simulink model "Sim_Multi"  (R2023a)
settings: Solver=FixedStepAuto  StartTime=0.0  StopTime=20  FixedStep=t_sim  MaxStep=t_control  RelTol=1e-5  EnableMultiTasking=on
InitFcn:
  | %--------------------------------------------------------------------------
  | %% Multirotor Dynamic Simulation Environment for the Testing of GNC Algorithms
  | % This simulation is part of the Master's thesis titled
  | % "A Modular Simulation Environment for the Improved Dynamic Simulation of
  | % Multirotor Unmanned Aerial Vehicles",
  | % submitted to the University of Illinois at Urbana-Champaign in May 2016.
  | % The thesis itself can be found here: http://hdl.handle.net/2142/90660
  | % Jan Vervoorst, vervoors@illinois.edu
  | % University of Illinois 2015/16
  | %--------------------------------------------------------------------------
  | %% Initialization routine for the Simulink simulation file Sim_Multi.slx
  | %--------------------------------------------------------------------------
  | clear all;close all;clc
  | %--------------------------------------------------------------------------
  | t_control = 1/500;          % Controller/state estimation frequency 500Hz [s]
  | t_sim = t_control/2;        % Simulation frequency 1000Hz [s]
  | sim_time = 10.0;            % Duration of simulation [sec]
  | r2d = 180/pi;               % Conversion factor radians to degrees [deg/rad]
  | d2r = pi/180;               % Conversion factor degrees to radians [rad/deg]
  | g = 9.80665;                % Acceleration of gravity [m/s^2]
  | rpm2radpersec = 2*pi/60;    % Conversion factor RPM to rad/sec [rad/(s*rpm)]
  | rho = 1.225;                % Density of air [kg/m^3]
  | %--------------------------------------------------------------------------
  | %%%%%%%%%%%%%%%%%%%%%%%%%%%%%%%%%%%%%%%%%%%%%%%%%%%%%%%%%%%%%%%%%%%%%%%%%%%
  | %               Quad specific configuration parameters                    %
  | %%%%%%%%%%%%%%%%%%%%%%%%%%%%%%%%%%%%%%%%%%%%%%%%%%%%%%%%%%%%%%%%%%%%%%%%%%%
  | % The coordinate system used in this model is defined as follows:
  | % X: pointing forward, Roll axis
  | % Y: pointing to the right, Pitch axis
  | % Z: pointing down, Yaw axis
  | % To define the geometry of the airframe, the following convention is used:
  | % - the base airframe is assumed to be somewhat symmetric
  | % - the CoG for the base airframe coincides with the geometric center in X/Y plane (but is shifted along Z axis)
  | % - the motor arm length in X/Y plane is defined as the distance to the geometric center of the base airframe
  | % - motor thrust is generated at the prop, which is offset a distance (along Z) from the geometric center
  | % - motor thrust vector may be misaligned from purely Z direction, so a set of rotation angles is given for each motor
  | % - real position of CoG is given as a position vector from geometric center
  | % - everything is expressed in body coordinate system described above
  | %%%%%%%%%%%%%%%%%%%%%%%%%%%%%%%%%%%%%%%%%%%%%%%%%%%%%%%%%%%%%%%%%%%%%%%%%%%
  | Noise_flag = 0;                 % Set to 1 for sensor/estimation noise, to 0 for no noise
  | Coriolis_correction = 1;        % Set to 1 to cancel omega x (J*omega) term in control law, 0 if not
  | Dyn_thrust = 1;                 % Set to 1 to engage dynamic thrust effects, to 0 to disengage
  | Blade_flapping = 1;             % Set to 1 to engage blade flapping effects, to 0 to disengage
  | %%%%%%%%%%%%%%%%%%%%%%%%%%%%%%%%
  | % Initial conditions
  | Att_init = [0;0;0] * d2r;       % Initial airframe attitude in Euler angles Roll/Pitch/Yaw for 6DOF block [deg]
  | omega_init = [0;0;0];           % Initial angular rates in Body frame for 6DOF block [rad/s]
  | Vb_init = [0;0;0];              % Initial velocity in Body frame for 6DOF block [m/s]
  | Xi_init = [0;0;0];              % Initial position in Inertial frame for 6DOF block [m]
  | rpm_init = 3104.5025852;        % Initial motor speed [rpm]
  | q_init = rpy2quat(Att_init);    % Compute the initial attitude quaternion
  | R_IB_init = rpy2rot(Att_init);  % Compute the initial rotation matrix R_IB
  | Vi_init = R_IB_init' * Vb_init; % Compute the initial velocity in Inertial axes
  | %%%%%%%%%%%%%%%%%%%%%%%%%%%%%%%%
  | % Parameters for aerodynamic drag computation
  | a = 0.060;                      % Surface area of airframe visible along the Body x axis [m^2]
  | b = 0.060;                      % Surface area of airframe visible along the Body y axis [m^2]
  | c = 0.060;                      % Surface area of airframe visible along the Body z axis [m^2]
  | C_D = 0.40;                     % Drag coefficient [dimensionless]
  | Surface_params = [a;b;c];       % Combine the surface area parameters
  | ... (+145 lines)
undefined symbols (not defined in the file or in its folder): DiscIntNeverNeededParam, rpy2quat, thrust2rpm
libraries: simulink x20
(part 2 of 4)

== system Sim_Multi/State Estimation, Sensors, Noise/State estimation/Normalize ==
  Input : Inport
  Divide : Product  Inputs=*/
  norm : Subsystem
  Output : Outport
  wires:
  Input/1 -> Divide/1, norm/1(u)
  norm/1(||u||) -> Divide/2
  Divide/1 -> Output/1

== system Sim_Multi/State Estimation, Sensors, Noise/State estimation/Quat noise ==
  Band-Limited White Noise : simulink/Sources/Band-Limited White Noise  Cov=t_sim*57.3*57.3/10000  Ts=t_sim*30  seed=[23099]
  Constant : Constant  Value=Noise_flag
  Constant1 : Constant  Value=0
  Gain2 : Gain  Gain=0.1
  Rate Transition1 : RateTransition  OutPortSampleTime=t_sim
  Switch : Switch  Criteria=u2 > Threshold  SaturateOnIntegerOverflow=off  InputSameDT=off
  Noise : Outport
  wires:
  Band-Limited White Noise/1 -> Gain2/1
  Switch/1 -> Noise/1
  Constant/1 -> Switch/2
  Constant1/1 -> Switch/3
  Gain2/1 -> Rate Transition1/1
  Rate Transition1/1 -> Switch/1

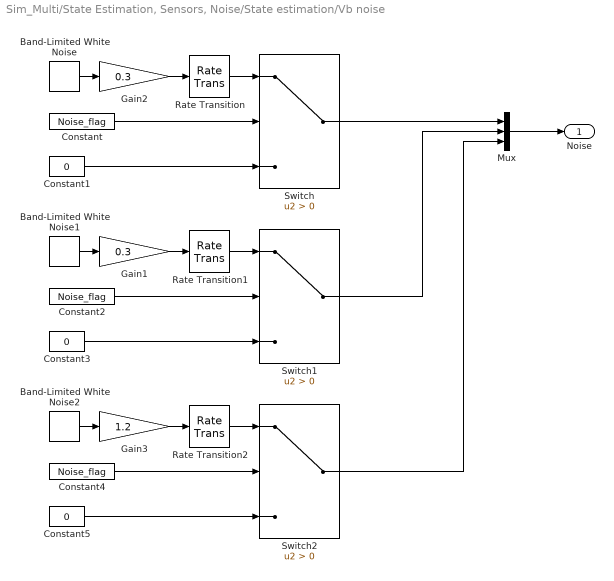
== system Sim_Multi/State Estimation, Sensors, Noise/State estimation/Vb noise ==
  Band-Limited White Noise : simulink/Sources/Band-Limited White Noise  Cov=t_sim*57.3*57.3/10000  Ts=t_sim*10  seed=[21234]
  Band-Limited White Noise1 : simulink/Sources/Band-Limited White Noise  Cov=t_sim*57.3*57.3/10000  Ts=t_sim*10  seed=[21234]
  Band-Limited White Noise2 : simulink/Sources/Band-Limited White Noise  Cov=t_sim*57.3*57.3/10000  Ts=t_sim*10  seed=[21234]
  Constant : Constant  Value=Noise_flag
  Constant1 : Constant  Value=0
  Constant2 : Constant  Value=Noise_flag
  Constant3 : Constant  Value=0
  Constant4 : Constant  Value=Noise_flag
  Constant5 : Constant  Value=0
  Gain1 : Gain  Gain=0.3
  Gain2 : Gain  Gain=0.3
  Gain3 : Gain  Gain=1.2
  Mux : Mux  Inputs=3
  Rate Transition : RateTransition  OutPortSampleTime=t_sim
  Rate Transition1 : RateTransition  OutPortSampleTime=t_sim
  Rate Transition2 : RateTransition  OutPortSampleTime=t_sim
  Switch : Switch  Criteria=u2 > Threshold  SaturateOnIntegerOverflow=off  InputSameDT=off
  Switch1 : Switch  Criteria=u2 > Threshold  SaturateOnIntegerOverflow=off  InputSameDT=off
  Switch2 : Switch  Criteria=u2 > Threshold  SaturateOnIntegerOverflow=off  InputSameDT=off
  Noise : Outport
  wires:
  Band-Limited White Noise/1 -> Gain2/1
  Constant/1 -> Switch/2
  Constant1/1 -> Switch/3
  Gain2/1 -> Rate Transition/1
  Rate Transition/1 -> Switch/1
  Switch/1 -> Mux/1
  Mux/1 -> Noise/1
  Band-Limited White Noise1/1 -> Gain1/1
  Constant2/1 -> Switch1/2
  Constant3/1 -> Switch1/3
  Gain1/1 -> Rate Transition1/1
  Rate Transition1/1 -> Switch1/1
  Band-Limited White Noise2/1 -> Gain3/1
  Constant4/1 -> Switch2/2
  Constant5/1 -> Switch2/3
  Gain3/1 -> Rate Transition2/1
  Rate Transition2/1 -> Switch2/1
  Switch1/1 -> Mux/2
  Switch2/1 -> Mux/3

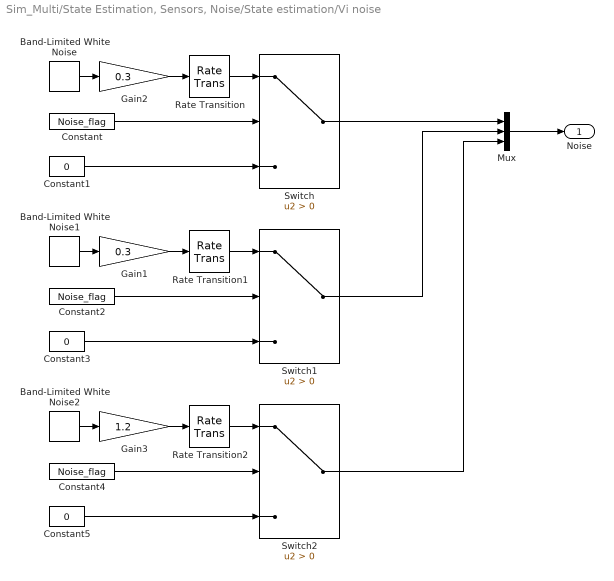
== system Sim_Multi/State Estimation, Sensors, Noise/State estimation/Vi noise ==
  Band-Limited White Noise : simulink/Sources/Band-Limited White Noise  Cov=t_sim*57.3*57.3/10000  Ts=t_sim*10  seed=[23888]
  Band-Limited White Noise1 : simulink/Sources/Band-Limited White Noise  Cov=t_sim*57.3*57.3/10000  Ts=t_sim*10  seed=[23888]
  Band-Limited White Noise2 : simulink/Sources/Band-Limited White Noise  Cov=t_sim*57.3*57.3/10000  Ts=t_sim*10  seed=[23888]
  Constant : Constant  Value=Noise_flag
  Constant1 : Constant  Value=0
  Constant2 : Constant  Value=Noise_flag
  Constant3 : Constant  Value=0
  Constant4 : Constant  Value=Noise_flag
  Constant5 : Constant  Value=0
  Gain1 : Gain  Gain=0.3
  Gain2 : Gain  Gain=0.3
  Gain3 : Gain  Gain=1.2
  Mux : Mux  Inputs=3
  Rate Transition : RateTransition  OutPortSampleTime=t_sim
  Rate Transition1 : RateTransition  OutPortSampleTime=t_sim
  Rate Transition2 : RateTransition  OutPortSampleTime=t_sim
  Switch : Switch  Criteria=u2 > Threshold  SaturateOnIntegerOverflow=off  InputSameDT=off
  Switch1 : Switch  Criteria=u2 > Threshold  SaturateOnIntegerOverflow=off  InputSameDT=off
  Switch2 : Switch  Criteria=u2 > Threshold  SaturateOnIntegerOverflow=off  InputSameDT=off
  Noise : Outport
  wires:
  Band-Limited White Noise/1 -> Gain2/1
  Constant/1 -> Switch/2
  Constant1/1 -> Switch/3
  Gain2/1 -> Rate Transition/1
  Rate Transition/1 -> Switch/1
  Switch/1 -> Mux/1
  Mux/1 -> Noise/1
  Band-Limited White Noise1/1 -> Gain1/1
  Constant2/1 -> Switch1/2
  Constant3/1 -> Switch1/3
  Gain1/1 -> Rate Transition1/1
  Rate Transition1/1 -> Switch1/1
  Band-Limited White Noise2/1 -> Gain3/1
  Constant4/1 -> Switch2/2
  Constant5/1 -> Switch2/3
  Gain3/1 -> Rate Transition2/1
  Rate Transition2/1 -> Switch2/1
  Switch1/1 -> Mux/2
  Switch2/1 -> Mux/3

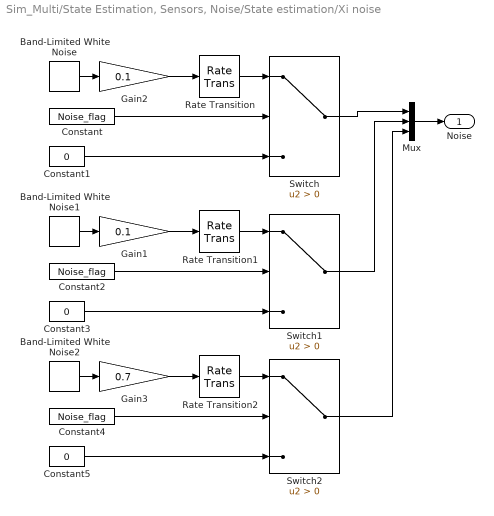
== system Sim_Multi/State Estimation, Sensors, Noise/State estimation/Xi noise ==
  Band-Limited White Noise : simulink/Sources/Band-Limited White Noise  Cov=t_sim*57.3*57.3/10000  Ts=t_sim*20  seed=[23559]
  Band-Limited White Noise1 : simulink/Sources/Band-Limited White Noise  Cov=t_sim*57.3*57.3/10000  Ts=t_sim*20  seed=[23559]
  Band-Limited White Noise2 : simulink/Sources/Band-Limited White Noise  Cov=t_sim*57.3*57.3/10000  Ts=t_sim*20  seed=[23559]
  Constant : Constant  Value=Noise_flag
  Constant1 : Constant  Value=0
  Constant2 : Constant  Value=Noise_flag
  Constant3 : Constant  Value=0
  Constant4 : Constant  Value=Noise_flag
  Constant5 : Constant  Value=0
  Gain1 : Gain  Gain=0.1
  Gain2 : Gain  Gain=0.1
  Gain3 : Gain  Gain=0.7
  Mux : Mux  Inputs=3
  Rate Transition : RateTransition  OutPortSampleTime=t_sim
  Rate Transition1 : RateTransition  OutPortSampleTime=t_sim
  Rate Transition2 : RateTransition  OutPortSampleTime=t_sim
  Switch : Switch  Criteria=u2 > Threshold  SaturateOnIntegerOverflow=off  InputSameDT=off
  Switch1 : Switch  Criteria=u2 > Threshold  SaturateOnIntegerOverflow=off  InputSameDT=off
  Switch2 : Switch  Criteria=u2 > Threshold  SaturateOnIntegerOverflow=off  InputSameDT=off
  Noise : Outport
  wires:
  Band-Limited White Noise/1 -> Gain2/1
  Constant/1 -> Switch/2
  Constant1/1 -> Switch/3
  Gain2/1 -> Rate Transition/1
  Mux/1 -> Noise/1
  Switch/1 -> Mux/1
  Band-Limited White Noise1/1 -> Gain1/1
  Constant2/1 -> Switch1/2
  Constant3/1 -> Switch1/3
  Gain1/1 -> Rate Transition1/1
  Band-Limited White Noise2/1 -> Gain3/1
  Constant4/1 -> Switch2/2
  Constant5/1 -> Switch2/3
  Gain3/1 -> Rate Transition2/1
  Switch1/1 -> Mux/2
  Switch2/1 -> Mux/3
  Rate Transition/1 -> Switch/1
  Rate Transition1/1 -> Switch1/1
  Rate Transition2/1 -> Switch2/1

== system Sim_Multi/multirotor/6DOF model/Body to Inertial ==
  V_b : Inport
  DCM_ib : Inport  Port=2
  Math Function2 : Math  Operator=transpose  SignedPower=on
  Product : Product  Multiplication=Matrix(*)
  Reshape : Reshape  OutputDimensionality=Column vector (2-D)
  Reshape1 : Reshape  OutputDimensionality=Column vector (2-D)
  V_i : Outport
  wires:
  Reshape/1 -> Product/2
  Product/1 -> Reshape1/1
  DCM_ib/1 -> Math Function2/1
  Reshape1/1 -> V_i/1
  V_b/1 -> Reshape/1
  Math Function2/1 -> Product/1  "DCM_bi"

== system Sim_Multi/multirotor/6DOF model/Body to Inertial1 ==
  a_b : Inport
  DCM_ib : Inport  Port=2
  Math Function2 : Math  Operator=transpose  SignedPower=on
  Product : Product  Multiplication=Matrix(*)
  Reshape : Reshape  OutputDimensionality=Column vector (2-D)
  Reshape1 : Reshape  OutputDimensionality=Column vector (2-D)
  a_i : Outport
  wires:
  Reshape/1 -> Product/2
  Product/1 -> Reshape1/1
  DCM_ib/1 -> Math Function2/1
  Reshape1/1 -> a_i/1
  a_b/1 -> Reshape/1
  Math Function2/1 -> Product/1  "DCM_bi"

== system Sim_Multi/multirotor/6DOF model/Calculate omega_dot ==
  omega [rad/s] : Inport
  Inertia [kgm^2] : Inport  Port=2
  Moments [Nm] : Inport  Port=3
  Cross Product omega x (J * omega) : Subsystem
  Product : Product  Inputs=/*  Multiplication=Matrix(*)
  Reshape : Reshape  OutputDimensionality=Column vector (2-D)
  "Reshape " : Reshape  OutputDimensionality=Column vector (2-D)
  Subsystem : Subsystem
  Sum1 : Sum  Inputs=-+|
  omega_dot [rad/s^2] : Outport
  wires:
  Inertia [kgm^2]/1 -> Product/1, Subsystem/2(J)
  omega [rad/s]/1 -> Cross Product omega x (J * omega)/1(omega), Subsystem/1(omega)
  Subsystem/1(J * omega) -> Cross Product omega x (J * omega)/2(J * omega)
  Cross Product omega x (J * omega)/1(omega x (J * omega)) -> Reshape/1
  Product/1 -> "Reshape "/1
  "Reshape "/1 -> omega_dot [rad/s^2]/1
  Moments [Nm]/1 -> Sum1/2
  Reshape/1 -> Sum1/1
  Sum1/1 -> Product/2

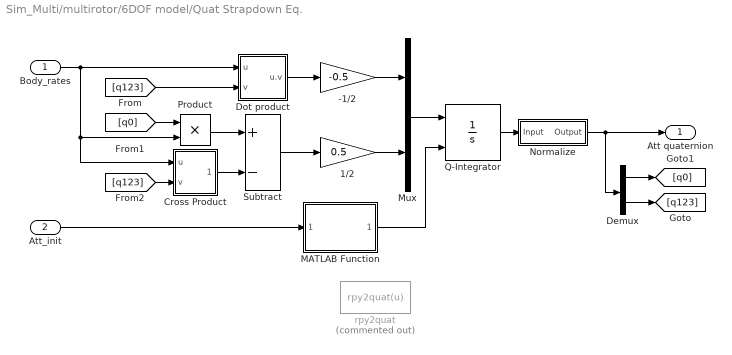
== system Sim_Multi/multirotor/6DOF model/Quat Strapdown Eq. ==
  Body_rates : Inport
  Att_init : Inport  Port=2
  -1/2 : Gain  Gain=-0.5
  1/2 : Gain  Gain=0.5
  Cross Product : Subsystem
  Demux : Demux  Outputs=[1 3]
  Dot product : Subsystem
  MATLAB Function : MATLAB Function  TreatAsAtomicUnit=on
  Mux : Mux  Inputs=[1 3]
  Normalize : Subsystem
  Product : Product  RndMeth=Zero
  Q-Integrator : Integrator  InitialConditionSource=external  InitialCondition=[1 0 0 0]
  Subtract : Sum  Inputs=+-
  rpy2quat : MATLABFcn  Commented=on  MATLABFcn=rpy2quat(u)  OutputDimensions=4
  Att quaternion : Outport
  wires:
  Dot product/1(u.v) -> -1/2/1
  -1/2/1 -> Mux/1
  Body_rates/1 -> Dot product/1(u), Cross Product/1(u), Product/2
  Q-Integrator/1 -> Normalize/1(Input)
  [q123] -> Dot product/2(v)
  Product/1 -> Subtract/1
  Cross Product/1(u x v) -> Subtract/2
  [q0] -> Product/1
  [q123] -> Cross Product/2(v)
  Subtract/1 -> 1/2/1
  1/2/1 -> Mux/2
  Demux/1 -> [q0]
  Demux/2 -> [q123]
  Normalize/1(Output) -> Demux/1, Att quaternion/1
  Mux/1 -> Q-Integrator/1
  MATLAB Function/1(quat_output) -> Q-Integrator/2
  Att_init/1 -> MATLAB Function/1(quat_input)

== system Sim_Multi/multirotor/6DOF model/Quat to Euler ==
  Quaternion q : Inport
  Fcn : Fcn  Expr=2*(u(3)*u(4)+u(1)*u(2))
  Fcn1 : Fcn  Expr=2*(u(2)*u(4)-u(1)*u(3))
  Fcn2 : Fcn  Expr=2*(u(2)*u(3)+u(1)*u(4))
  Fcn3 : Fcn  Expr=u(1)*u(1)-u(2)*u(2)-u(3)*u(3)+u(4)*u(4)
  Fcn4 : Fcn  Expr=u(1)*u(1)+u(2)*u(2)-u(3)*u(3)-u(4)*u(4)
  Gain : Gain  Gain=-1
  Reshape : Reshape  OutputDimensionality=Column vector (2-D)
  Trigonometric Function : Trigonometry  Operator=asin
  Trigonometric Function1 : Trigonometry  Operator=atan2
  Trigonometric Function2 : Trigonometry  Operator=atan2
  Vector Concatenate : Concatenate  NumInputs=3
  Euler [rad] : Outport
  wires:
  Fcn1/1 -> Trigonometric Function/1
  Trigonometric Function/1 -> Gain/1
  Fcn/1 -> Trigonometric Function1/1
  Fcn3/1 -> Trigonometric Function1/2
  Fcn2/1 -> Trigonometric Function2/1
  Fcn4/1 -> Trigonometric Function2/2
  Trigonometric Function1/1 -> Vector Concatenate/1
  Gain/1 -> Vector Concatenate/2
  Trigonometric Function2/1 -> Vector Concatenate/3
  Quaternion q/1 -> Fcn4/1, Fcn2/1, Fcn/1, Fcn3/1, Fcn1/1
  Vector Concatenate/1 -> Reshape/1
  Reshape/1 -> Euler [rad]/1

== system Sim_Multi/multirotor/6DOF model/Quat to Rotation Matrix ==
  Quaternion q : Inport
  Subsystem : Subsystem
  Subsystem1 : Subsystem
  Subsystem2 : Subsystem
  Subsystem3 : Subsystem
  Subsystem4 : Subsystem
  Subsystem5 : Subsystem
  Subsystem6 : Subsystem
  Subsystem7 : Subsystem
  Subsystem8 : Subsystem
  Subsystem9 : Subsystem
  DCM_ib : Outport
  wires:
  Quaternion q/1 -> Subsystem2/1(q), Subsystem8/1(q), Subsystem7/1(q), Subsystem6/1(q), Subsystem1/1(q), Subsystem5/1(q), Subsystem4/1(q), Subsystem3/1(q), Subsystem/1(q)
  Subsystem/1(C_11) -> Subsystem9/1(C_11)
  Subsystem3/1(C_12) -> Subsystem9/2(C_12)
  Subsystem4/1(C_13) -> Subsystem9/3(C_13)
  Subsystem5/1(C_21) -> Subsystem9/4(C_21)
  Subsystem1/1(C_22) -> Subsystem9/5(C_22)
  Subsystem2/1(C_33) -> Subsystem9/9(C_33)
  Subsystem8/1(C_32) -> Subsystem9/8(C_32)
  Subsystem7/1(C_31) -> Subsystem9/7(C_31)
  Subsystem6/1(C_23) -> Subsystem9/6(C_23)
  Subsystem9/1(DCM_ib) -> DCM_ib/1

== system Sim_Multi/multirotor/6DOF model/omega x V_b ==
  V_b : Inport
  omega : Inport  Port=2
  Subsystem : Subsystem
  Subsystem1 : Subsystem
  Sum : Sum  Inputs=+|-
  omega x V_b : Outport
  wires:
  Sum/1 -> omega x V_b/1
  omega/1 -> Subsystem1/1(u), Subsystem/1(u)
  V_b/1 -> Subsystem/2(v), Subsystem1/2(v)
  Subsystem/1(Positive elements) -> Sum/1
  Subsystem1/1(Negative elements) -> Sum/2

== system Sim_Multi/multirotor/Force//Moment computation/Compute aerodynamic drag of the airframe in Body axes ==
  note: Aerodynamic drag force acting on the airframe
      | The assumption is that the surface area of the airframe from different directions
      | can be described by an ellipsoid. Then the 'acting 'surface area is in the direction
      | of the airspeed vector and can be computed by scaling the airspeed vector so that
      | it points onto the surface of the ellipsoid.
  6DOF dynamics : Inport
  Dynamic parameters : Inport  Port=2
  Aerodynamic drag force : Subsystem
  Bus Selector2 : BusSelector  OutputSignals=V_b,DCM_ib
  Bus Selector3 : BusSelector  OutputSignals=Wind_i,Surface_params
  Total airspeed (Body axes) : Subsystem
  Drag force : Outport
  wires:
  Aerodynamic drag force/1(Drag force (Body axes)) -> Drag force/1
  6DOF dynamics/1 -> Bus Selector2/1
  Dynamic parameters/1 -> Bus Selector3/1
  Bus Selector3/2 -> Aerodynamic drag force/2(Surface_params)  "<Surface_params>"
  Bus Selector2/1 -> Total airspeed (Body axes)/1(V_b)  "<V_b>"
  Bus Selector2/2 -> Total airspeed (Body axes)/2(DCM_ib)  "<DCM_ib>"
  Bus Selector3/1 -> Total airspeed (Body axes)/3(Wind_i)  "<Wind_i>"
  Total airspeed (Body axes)/1(Airspeed (Body)) -> Aerodynamic drag force/1(Airspeed (Body axes))

== system Sim_Multi/multirotor/Force//Moment computation/Compute force of gravity in Body axes ==
  note: Force of gravity acting on the airframe
  6DOF dynamics : Inport
  Dynamic parameters : Inport  Port=2
  Bus Selector : BusSelector  OutputSignals=DCM_ib
  Bus Selector1 : BusSelector  OutputSignals=mass_real
  Gravity (Inertial axes) : Constant  Value=[0;0;g]
  Product : Product  Multiplication=Matrix(*)  InputSameDT=on  SaturateOnIntegerOverflow=on  OutDataTypeStr=Inherit: Same as first input
  Product1 : Product
  Reshape : Reshape  OutputDimensionality=Column vector (2-D)
  Gravity force : Outport
  wires:
  Gravity (Inertial axes)/1 -> Product1/1
  Product1/1 -> Product/2  "Force of gravity (Inertial axes)"
  Product/1 -> Reshape/1  "Force of gravity (Body axes)"
  Reshape/1 -> Gravity force/1
  6DOF dynamics/1 -> Bus Selector/1
  Dynamic parameters/1 -> Bus Selector1/1
  Bus Selector1/1 -> Product1/2  "<mass_real>"
  Bus Selector/1 -> Product/1  "<DCM_ib>"

== system Sim_Multi/multirotor/Force//Moment computation/Forces and moments generated by spinning propellers ==
  note: Computation of forces and moments for each actuator specified in the initialization routine
  RPM_commands : Inport
  Dynamic parameters : Inport  Port=2
  6DOF dynamics : Inport  Port=3
  Bus Selector : BusSelector  OutputSignals=omega,V_b,DCM_ib
  Bus Selector1 : BusSelector  OutputSignals=Wind_i,MotorMatrix_real,CoG_real
  For Each Subsystem : Subsystem  TreatAsAtomicUnit=on
  Reshape : Reshape  OutputDimensionality=Column vector (2-D)
  Sum of Elements : Sum  Inputs=+  CollapseMode=Specified dimension  CollapseDim=2
  Sum of Elements1 : Sum  Inputs=+  CollapseMode=Specified dimension  CollapseDim=2
  To Workspace : ToWorkspace  VariableName=rpm_motor  SaveFormat=Structure With Time  SampleTime=-1
      settings: Save2DSignal=2-D array (concatenate along first dimension)
  Total airspeed (Body axes) : Subsystem
  Motor moments : Outport
  Motor forces : Outport  Port=2
  motor_RPM : Outport  Port=3
  tag scope: RPM_motor=global
  wires:
  For Each Subsystem/1(Motor_force) -> Sum of Elements/1
  For Each Subsystem/2(Motor_moment) -> Sum of Elements1/1
  Sum of Elements/1 -> Motor forces/1
  Sum of Elements1/1 -> Motor moments/1
  RPM_commands/1 -> For Each Subsystem/1(RPM_commands)
  6DOF dynamics/1 -> Bus Selector/1
  Bus Selector/1 -> For Each Subsystem/2(Body_rates)  "<omega>"
  Dynamic parameters/1 -> Bus Selector1/1
  Bus Selector1/2 -> For Each Subsystem/4(MotorMatrix_real)  "<MotorMatrix_real>"
  Bus Selector1/3 -> For Each Subsystem/5(CoG_real)  "<CoG_real>"
  Bus Selector/2 -> Total airspeed (Body axes)/1(V_b)  "<V_b>"
  Bus Selector/3 -> Total airspeed (Body axes)/2(DCM_ib)  "<DCM_ib>"
  Bus Selector1/1 -> Total airspeed (Body axes)/3(Wind_i)  "<Wind_i>"
  Total airspeed (Body axes)/1(Airspeed (Body)) -> For Each Subsystem/3(Airspeed (Body))
  For Each Subsystem/3(RPM_motor) -> Reshape/1
  Reshape/1 -> To Workspace/1, motor_RPM/1, [RPM_motor]

== system Sim_Multi/Controller/Controller Structure/Inner-loop control only/Conversion stick values to rate commands ==
  Sticks/Throttle cmd : Inport
  Constant : Constant  Value=thrust_offset
  Demux8 : Demux  Outputs=[3 1]
  Mux3 : Mux  Inputs=2
  Sum4 : Sum  Inputs=|++
  Unit conversion [stick value] to [N] : Gain  Gain=thrust_gain
  Unit conversion [stick value] to [rad/s] : Gain  Gain=MaxRate_cmd/500
  Rates/Throttle cmd : Outport
  wires:
  Sticks/Throttle cmd/1 -> Demux8/1
  Demux8/1 -> Unit conversion [stick value] to [rad/s]/1
  Unit conversion [stick value] to [N]/1 -> Sum4/1
  Constant/1 -> Sum4/2
  Demux8/2 -> Unit conversion [stick value] to [N]/1  "Throttle cmd"
  Sum4/1 -> Mux3/2  "Throttle command (thrust value)"
  Mux3/1 -> Rates/Throttle cmd/1
  Unit conversion [stick value] to [rad/s]/1 -> Mux3/1

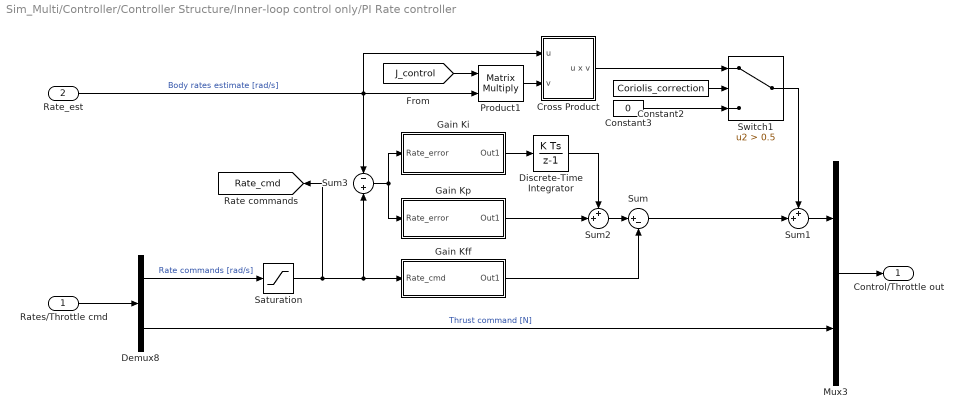
== system Sim_Multi/Controller/Controller Structure/Inner-loop control only/PI Rate controller ==
  Rates/Throttle cmd : Inport
  Rate_est : Inport  Port=2
  Constant2 : Constant  Value=Coriolis_correction
  Constant3 : Constant  Value=0
  Cross Product : Subsystem
  Demux8 : Demux  Outputs=[3 1]
  Discrete-Time Integrator : DiscreteIntegrator  SampleTime=t_control  ICPrevOutput=DiscIntNeverNeededParam  ICPrevScaledInput=DiscIntNeverNeededParam
  Gain Kff : Subsystem
  Gain Ki : Subsystem
  Gain Kp : Subsystem
  Mux3 : Mux  Inputs=2
  Product1 : Product  Multiplication=Matrix(*)  RndMeth=Zero  SampleTime=t_control
  Saturation : Saturate  UpperLimit=MaxRate_cmd  LowerLimit=-MaxRate_cmd
  Sum : Sum  Inputs=|+-
  Sum1 : Sum  Inputs=++|
  Sum2 : Sum  Inputs=++|
  Sum3 : Sum  Inputs=-|+
  Switch1 : Switch  Criteria=u2 > Threshold  Threshold=0.5  SampleTime=t_control  SaturateOnIntegerOverflow=off  InputSameDT=off
  Control/Throttle out : Outport
  tag scope: Rate_cmd=global
  wires:
  Rate_est/1 -> Product1/2, Sum3/1, Cross Product/1(u)  "Body rates estimate [rad/s]"
  Mux3/1 -> Control/Throttle out/1
  Rates/Throttle cmd/1 -> Demux8/1
  Gain Ki/1(Out1) -> Discrete-Time Integrator/1
  Discrete-Time Integrator/1 -> Sum2/1
  Gain Kp/1(Out1) -> Sum2/2
  [J_control] -> Product1/1
  Product1/1 -> Cross Product/2(v)
  Sum1/1 -> Mux3/1
  Demux8/1 -> Saturation/1  "Rate commands [rad/s]"
  Sum3/1 -> Gain Kp/1(Rate_error), Gain Ki/1(Rate_error)
  Sum/1 -> Sum1/2
  Sum2/1 -> Sum/1
  Gain Kff/1(Out1) -> Sum/2
  Demux8/2 -> Mux3/2  "Thrust command [N]"
  Constant2/1 -> Switch1/2
  Cross Product/1(u x v) -> Switch1/1
  Constant3/1 -> Switch1/3
  Switch1/1 -> Sum1/1
  Saturation/1 -> [Rate_cmd], Sum3/2, Gain Kff/1(Rate_cmd)

== system Sim_Multi/State Estimation, Sensors, Noise/State estimation/Normalize/norm ==
  u : Inport
  Complex to Real-Imag : ComplexToRealImag  Output=Real
  Sqrt : Sqrt
  dot_product : Subsystem
  ||u|| : Outport
  wires:
  u/1 -> dot_product/1(u), dot_product/2(v)
  dot_product/1(u.v) -> Sqrt/1
  Sqrt/1 -> Complex to Real-Imag/1
  Complex to Real-Imag/1 -> ||u||/1

== system Sim_Multi/multirotor/6DOF model/Calculate omega_dot/Cross Product omega x (J * omega) ==
  omega : Inport
  J * omega : Inport  Port=2
  Subsystem : Subsystem
  Subsystem1 : Subsystem
  Sum : Sum  Inputs=+|-
  omega x (J * omega) : Outport
  wires:
  Sum/1 -> omega x (J * omega)/1
  omega/1 -> Subsystem1/1(u), Subsystem/1(u)
  J * omega/1 -> Subsystem/2(v), Subsystem1/2(v)
  Subsystem/1(Positive elements) -> Sum/1
  Subsystem1/1(Negative elements) -> Sum/2

== system Sim_Multi/multirotor/6DOF model/Calculate omega_dot/Subsystem ==
  omega : Inport
  J : Inport  Port=2
  Product : Product  Multiplication=Matrix(*)
  Reshape : Reshape  OutputDimensionality=Column vector (2-D)
  Reshape1 : Reshape  OutputDimensionality=Column vector (2-D)
  J * omega : Outport
  wires:
  Reshape1/1 -> J * omega/1
  Product/1 -> Reshape1/1
  J/1 -> Product/1
  Reshape/1 -> Product/2
  omega/1 -> Reshape/1

== system Sim_Multi/multirotor/6DOF model/Quat Strapdown Eq./Cross Product ==
  u : Inport
  v : Inport  Port=2
  Subsystem : Subsystem
  Subsystem1 : Subsystem
  Sum : Sum  Inputs=+|-
  u x v : Outport
  wires:
  Sum/1 -> u x v/1
  u/1 -> Subsystem1/1(u), Subsystem/1(u)
  v/1 -> Subsystem1/2(v), Subsystem/2(v)
  Subsystem/1(Positive elements) -> Sum/1
  Subsystem1/1(Negative elements) -> Sum/2

== system Sim_Multi/multirotor/6DOF model/Quat Strapdown Eq./Dot product ==
  u : Inport
  v : Inport  Port=2
  Product : Product  Multiplication=Matrix(*)  RndMeth=Zero
  Reshape : Reshape  OutputDimensionality=Column vector (2-D)
  Reshape1 : Reshape  OutputDimensionality=Column vector (2-D)
  transpose : Math  Operator=transpose  SignedPower=on
  u.v : Outport
  wires:
  v/1 -> Reshape1/1
  u/1 -> Reshape/1
  Reshape/1 -> transpose/1
  transpose/1 -> Product/1
  Reshape1/1 -> Product/2
  Product/1 -> u.v/1

== system Sim_Multi/multirotor/6DOF model/Quat Strapdown Eq./Normalize ==
  Input : Inport
  Divide : Product  Inputs=*/
  norm : Subsystem
  Output : Outport
  wires:
  Input/1 -> Divide/1, norm/1(u)
  norm/1(||u||) -> Divide/2
  Divide/1 -> Output/1

== system Sim_Multi/multirotor/6DOF model/Quat to Rotation Matrix/Subsystem ==
  q : Inport
  Add : Sum  Inputs=++--
  Demux : Demux
  Product{,2..4} (4 alike) : Product
  C_11 : Outport
  wires:
  Product2/1 -> Add/2
  Product4/1 -> Add/4
  Add/1 -> C_11/1
  Demux/2 -> Product2/2, Product2/1
  Product3/1 -> Add/3
  Demux/3 -> Product3/2, Product3/1
  Demux/1 -> Product/2, Product/1
  q/1 -> Demux/1
  Product/1 -> Add/1
  Demux/4 -> Product4/2, Product4/1

== system Sim_Multi/multirotor/6DOF model/Quat to Rotation Matrix/Subsystem1 ==
  q : Inport
  Add : Sum  Inputs=+-+-
  Demux : Demux
  Product{,2..4} (4 alike) : Product
  C_22 : Outport
  wires:
  Product2/1 -> Add/2
  Product4/1 -> Add/4
  Add/1 -> C_22/1
  Demux/2 -> Product2/2, Product2/1
  Product3/1 -> Add/3
  Demux/3 -> Product3/2, Product3/1
  Demux/1 -> Product/2, Product/1
  q/1 -> Demux/1
  Product/1 -> Add/1
  Demux/4 -> Product4/2, Product4/1

== system Sim_Multi/multirotor/6DOF model/Quat to Rotation Matrix/Subsystem2 ==
  q : Inport
  Add : Sum  Inputs=+--+
  Demux : Demux
  Product{,2..4} (4 alike) : Product
  C_33 : Outport
  wires:
  Product2/1 -> Add/2
  Product4/1 -> Add/4
  Add/1 -> C_33/1
  Demux/2 -> Product2/2, Product2/1
  Product3/1 -> Add/3
  Demux/3 -> Product3/2, Product3/1
  Demux/1 -> Product/2, Product/1
  q/1 -> Demux/1
  Product/1 -> Add/1
  Demux/4 -> Product4/2, Product4/1

== system Sim_Multi/multirotor/6DOF model/Quat to Rotation Matrix/Subsystem3 ==
  q : Inport
  Add : Sum
  Demux : Demux
  Gain : Gain  Gain=2
  Product : Product
  Product2 : Product
  C_12 : Outport
  wires:
  Add/1 -> Gain/1
  q/1 -> Demux/1
  Demux/2 -> Product/1
  Demux/3 -> Product/2
  Demux/1 -> Product2/1
  Demux/4 -> Product2/2
  Product/1 -> Add/1
  Product2/1 -> Add/2
  Gain/1 -> C_12/1

== system Sim_Multi/multirotor/6DOF model/Quat to Rotation Matrix/Subsystem4 ==
  q : Inport
  Add : Sum  Inputs=+-
  Demux : Demux
  Gain : Gain  Gain=2
  Product : Product
  Product2 : Product
  C_13 : Outport
  wires:
  Add/1 -> Gain/1
  q/1 -> Demux/1
  Product/1 -> Add/1
  Product2/1 -> Add/2
  Gain/1 -> C_13/1
  Demux/2 -> Product/1
  Demux/4 -> Product/2
  Demux/1 -> Product2/1
  Demux/3 -> Product2/2

== system Sim_Multi/multirotor/6DOF model/Quat to Rotation Matrix/Subsystem5 ==
  q : Inport
  Add : Sum  Inputs=+-
  Demux : Demux
  Gain : Gain  Gain=2
  Product : Product
  Product2 : Product
  C_21 : Outport
  wires:
  Add/1 -> Gain/1
  q/1 -> Demux/1
  Product/1 -> Add/1
  Product2/1 -> Add/2
  Gain/1 -> C_21/1
  Demux/2 -> Product/1
  Demux/3 -> Product/2
  Demux/1 -> Product2/1
  Demux/4 -> Product2/2

== system Sim_Multi/multirotor/6DOF model/Quat to Rotation Matrix/Subsystem6 ==
  q : Inport
  Add : Sum
  Demux : Demux
  Gain : Gain  Gain=2
  Product : Product
  Product2 : Product
  C_23 : Outport
  wires:
  Add/1 -> Gain/1
  q/1 -> Demux/1
  Product/1 -> Add/1
  Product2/1 -> Add/2
  Gain/1 -> C_23/1
  Demux/3 -> Product/1
  Demux/4 -> Product/2
  Demux/1 -> Product2/1
  Demux/2 -> Product2/2

== system Sim_Multi/multirotor/6DOF model/Quat to Rotation Matrix/Subsystem7 ==
  q : Inport
  Add : Sum
  Demux : Demux
  Gain : Gain  Gain=2
  Product : Product
  Product2 : Product
  C_31 : Outport
  wires:
  Add/1 -> Gain/1
  q/1 -> Demux/1
  Product/1 -> Add/1
  Product2/1 -> Add/2
  Gain/1 -> C_31/1
  Demux/2 -> Product/1
  Demux/4 -> Product/2
  Demux/1 -> Product2/1
  Demux/3 -> Product2/2

== system Sim_Multi/multirotor/6DOF model/Quat to Rotation Matrix/Subsystem8 ==
  q : Inport
  Add : Sum  Inputs=+-
  Demux : Demux
  Gain : Gain  Gain=2
  Product : Product
  Product2 : Product
  C_32 : Outport
  wires:
  Add/1 -> Gain/1
  q/1 -> Demux/1
  Product/1 -> Add/1
  Product2/1 -> Add/2
  Gain/1 -> C_32/1
  Demux/3 -> Product/1
  Demux/4 -> Product/2
  Demux/1 -> Product2/1
  Demux/2 -> Product2/2

== system Sim_Multi/multirotor/6DOF model/Quat to Rotation Matrix/Subsystem9 ==
  C_11 : Inport  PortDimensions=1
  C_12 : Inport  Port=2  PortDimensions=1
  C_13 : Inport  Port=3  PortDimensions=1
  C_21 : Inport  Port=4  PortDimensions=1
  C_22 : Inport  Port=5  PortDimensions=1
  C_23 : Inport  Port=6  PortDimensions=1
  C_31 : Inport  Port=7  PortDimensions=1
  C_32 : Inport  Port=8  PortDimensions=1
  C_33 : Inport  Port=9  PortDimensions=1
  Reshape (9) to [3x3] column-major : Reshape  OutputDimensionality=Customize  OutputDimensions=[3,3]
  Vector Concatenate : Concatenate  NumInputs=9
  DCM_ib : Outport
  wires:
  C_33/1 -> Vector Concatenate/9
  C_22/1 -> Vector Concatenate/5
  Reshape (9) to [3x3] column-major/1 -> DCM_ib/1
  C_11/1 -> Vector Concatenate/1
  Vector Concatenate/1 -> Reshape (9) to [3x3] column-major/1
  C_32/1 -> Vector Concatenate/6
  C_31/1 -> Vector Concatenate/3
  C_21/1 -> Vector Concatenate/2
  C_13/1 -> Vector Concatenate/7
  C_12/1 -> Vector Concatenate/4
  C_23/1 -> Vector Concatenate/8

== system Sim_Multi/multirotor/6DOF model/omega x V_b/Subsystem ==
  u : Inport
  v : Inport  Port=2
  Demux : Demux  Outputs=3
  Demux1 : Demux  Outputs=3
  Mux : Mux  Inputs=3
  Product : Product
  Product1 : Product
  Product2 : Product
  Positive elements : Outport
  wires:
  Mux/1 -> Positive elements/1
  v/1 -> Demux1/1
  u/1 -> Demux/1
  Demux/2 -> Product/1
  Demux1/3 -> Product/2
  Demux/3 -> Product1/1
  Demux1/1 -> Product1/2
  Demux/1 -> Product2/1
  Demux1/2 -> Product2/2
  Product/1 -> Mux/1  "u2*v3"
  Product1/1 -> Mux/2  "u3*v1"
  Product2/1 -> Mux/3  "u1*v2"

== system Sim_Multi/multirotor/6DOF model/omega x V_b/Subsystem1 ==
  u : Inport
  v : Inport  Port=2
  Demux : Demux  Outputs=3
  Demux1 : Demux  Outputs=3
  Mux : Mux  Inputs=3
  Product : Product
  Product1 : Product
  Product2 : Product
  Negative elements : Outport
  wires:
  Mux/1 -> Negative elements/1
  v/1 -> Demux1/1
  u/1 -> Demux/1
  Product/1 -> Mux/1  "u3*v2"
  Product1/1 -> Mux/2  "u1*v3"
  Product2/1 -> Mux/3  "u2*v1"
  Demux/3 -> Product/1
  Demux1/2 -> Product/2
  Demux/1 -> Product1/1
  Demux1/3 -> Product1/2
  Demux/2 -> Product2/1
  Demux1/1 -> Product2/2

== system Sim_Multi/multirotor/Force//Moment computation/Compute aerodynamic drag of the airframe in Body axes/Aerodynamic drag force ==
  note: This block computes the surface area of the airframe that is visible in the direction of the airspeed.
      | Drag force is computed by the standard drag equation: 1/2*rho*u^2*C_D*A
  Airspeed (Body axes) : Inport
  Surface_params : Inport  Port=2
  If : If  IfExpression=u1 == 0
  Merge : Merge
  Nonzero airspeed : Subsystem  TreatAsAtomicUnit=on
  Zero airspeed : Subsystem  TreatAsAtomicUnit=on
  norm : Subsystem
  Drag force (Body axes) : Outport
  wires:
  If/1 -> Zero airspeed/Action
  Zero airspeed/1(Drag force) -> Merge/1
  Nonzero airspeed/1(Drag force) -> Merge/2
  If/2 -> Nonzero airspeed/Action
  Airspeed (Body axes)/1 -> norm/1(u), Nonzero airspeed/1(Airspeed (Body)), Zero airspeed/1(Airspeed)
  norm/1(||u||) -> If/1  "Airspeed magnitude"
  Merge/1 -> Drag force (Body axes)/1  "Force against direction of motion due to aerodynamic drag"
  Surface_params/1 -> Nonzero airspeed/2(Surface_params), Zero airspeed/2(Surface_params)

== system Sim_Multi/multirotor/Force//Moment computation/Compute aerodynamic drag of the airframe in Body axes/Total airspeed (Body axes) ==
  V_b : Inport
  DCM_ib : Inport  Port=2
  Wind_i : Inport  Port=3
  Inertial to Body : Subsystem
  Reshape : Reshape  OutputDimensionality=Column vector (2-D)
  Sum1 : Sum  Inputs=|+-
  Airspeed (Body) : Outport
  wires:
  DCM_ib/1 -> Inertial to Body/1(DCM_ib)
  Wind_i/1 -> Inertial to Body/2(Wind_i)
  Inertial to Body/1(Wind_b) -> Sum1/2  "Wind velocity (Body axes)"
  Reshape/1 -> Sum1/1
  V_b/1 -> Reshape/1
  Sum1/1 -> Airspeed (Body)/1  "True airspeed (Body axes)"

== system Sim_Multi/multirotor/Force//Moment computation/Forces and moments generated by spinning propellers/For Each Subsystem ==
  note: This subsystem computes all the forces and moments generated by each of the actuators.
      |
      | That includes dynamic thrust, blade flapping effects, gyroscopic moments, and others.
      | All forces and moments are computed as acting on the real center of gravity of the airframe,
      | which might change during the simulation due to failure cases or the dropping of cargo.
      |
      | Outputs are the total force and moment vectors for each one of the motors.
  RPM_commands : Inport  Partition=on  PartitionDimension=1  PartitionWidth=1  PartitionOffset=0
  Body_rates : Inport  Port=2
  Airspeed (Body) : Inport  Port=3
  MotorMatrix_real : Inport  Port=4  Partition=on  PartitionDimension=1  PartitionWidth=1  PartitionOffset=0
  CoG_real : Inport  Port=5
  Actuator dynamics : Subsystem
  Cross Product : Subsystem
  For Each : ForEach  DisableCoverage=on
  Leverarm vector from real CoG to each propeller (Body axes) : Subsystem
  Rate Transition : RateTransition  OutPortSampleTime=t_sim
  Sum1 : Sum  Inputs=|++
  Thrust/moment vector for each propeller (Body axes) : Subsystem
  Motor_force : Outport  ConcatenationDimension=2
  Motor_moment : Outport  Port=2  ConcatenationDimension=2
  RPM_motor : Outport  Port=3  ConcatenationDimension=2
  wires:
  Leverarm vector from real CoG to each propeller (Body axes)/1(Prop_vector) -> Cross Product/1(r), Thrust/moment vector for each propeller (Body axes)/1(Prop_vector)  "Leverarm vector from real CoG to propeller (Body axes)"
  MotorMatrix_real/1 -> Leverarm vector from real CoG to each propeller (Body axes)/1(MotorMatrix_real), Thrust/moment vector for each propeller (Body axes)/4(MotorMatrix_real), Actuator dynamics/1(MotorMatrix_real)
  Thrust/moment vector for each propeller (Body axes)/1(Thrust_vector (Body axes)) -> Motor_force/1  "Thrust force vector for each motor (Body axes)"
  Thrust/moment vector for each propeller (Body axes)/2(Motor_moments (Body axes)) -> Motor_moment/1  "Moment vector for each motor (Body axes)"
  RPM_commands/1 -> Rate Transition/1
  Body_rates/1 -> Thrust/moment vector for each propeller (Body axes)/3(Body_rates), Cross Product/2(omega)
  CoG_real/1 -> Leverarm vector from real CoG to each propeller (Body axes)/2(CoG_real)
  Cross Product/1(omega x r) -> Sum1/1  "Linear velocity at prop due to body angular rates (Body axes)"
  Airspeed (Body)/1 -> Sum1/2  "True linear velocity of airframe (including wind) (Body axes)"
  Sum1/1 -> Thrust/moment vector for each propeller (Body axes)/2(True airspeed)  "Total linear velocity at prop (Body axes)"
  Actuator dynamics/1(RPM_motor) -> RPM_motor/1, Thrust/moment vector for each propeller (Body axes)/5(RPM_motor)  "Actual motor RPM"
  Rate Transition/1 -> Actuator dynamics/2(RPM_command)

== system Sim_Multi/multirotor/Force//Moment computation/Forces and moments generated by spinning propellers/Total airspeed (Body axes) ==
  V_b : Inport
  DCM_ib : Inport  Port=2
  Wind_i : Inport  Port=3
  Inertial to Body : Subsystem
  Reshape : Reshape  OutputDimensionality=Column vector (2-D)
  Sum1 : Sum  Inputs=|+-
  Airspeed (Body) : Outport
  wires:
  DCM_ib/1 -> Inertial to Body/1(DCM_ib)
  Wind_i/1 -> Inertial to Body/2(Wind_i)
  Inertial to Body/1(Wind_b) -> Sum1/2  "Wind velocity (Body axes)"
  Sum1/1 -> Airspeed (Body)/1  "True airspeed (Body axes)"
  Reshape/1 -> Sum1/1
  V_b/1 -> Reshape/1

== system Sim_Multi/Controller/Controller Structure/Inner-loop control only/PI Rate controller/Cross Product ==
  u : Inport
  v : Inport  Port=2
  Subsystem : Subsystem
  Subsystem1 : Subsystem
  Sum : Sum  Inputs=+|-
  u x v : Outport
  wires:
  Sum/1 -> u x v/1
  u/1 -> Subsystem1/1(u), Subsystem/1(u)
  v/1 -> Subsystem1/2(v), Subsystem/2(v)
  Subsystem/1(Positive elements) -> Sum/1
  Subsystem1/1(Negative elements) -> Sum/2

== system Sim_Multi/Controller/Controller Structure/Inner-loop control only/PI Rate controller/Gain Kff ==
  Rate_cmd : Inport
  Constant1 : Constant  Value=Kff_1
  Create diagonal 3x3 matrix : Subsystem
  Product : Product  Multiplication=Matrix(*)  RndMeth=Zero  SampleTime=t_control
  Product1 : Product  Multiplication=Matrix(*)  RndMeth=Zero
  Out1 : Outport
  wires:
  [J_control] -> Product1/1
  Product1/1 -> Product/1
  Rate_cmd/1 -> Product/2
  Constant1/1 -> Create diagonal 3x3 matrix/1(Vector)
  Create diagonal 3x3 matrix/1(Matrix) -> Product1/2
  Product/1 -> Out1/1

== system Sim_Multi/Controller/Controller Structure/Inner-loop control only/PI Rate controller/Gain Ki ==
  Rate_error : Inport
  Constant1 : Constant  Value=Ki_1
  Create diagonal 3x3 matrix : Subsystem
  Product : Product  Multiplication=Matrix(*)  RndMeth=Zero  SampleTime=t_control
  Product1 : Product  Multiplication=Matrix(*)  RndMeth=Zero
  Out1 : Outport
  wires:
  [J_control] -> Product1/1
  Product1/1 -> Product/1
  Rate_error/1 -> Product/2
  Constant1/1 -> Create diagonal 3x3 matrix/1(Vector)
  Create diagonal 3x3 matrix/1(Matrix) -> Product1/2
  Product/1 -> Out1/1

== system Sim_Multi/Controller/Controller Structure/Inner-loop control only/PI Rate controller/Gain Kp ==
  Rate_error : Inport
  Constant1 : Constant  Value=Kp_1
  Create diagonal 3x3 matrix : Subsystem
  Product : Product  Multiplication=Matrix(*)  RndMeth=Zero  SampleTime=t_control
  Product1 : Product  Multiplication=Matrix(*)  RndMeth=Zero
  Out1 : Outport
  wires:
  [J_control] -> Product1/1
  Product1/1 -> Product/1
  Rate_error/1 -> Product/2
  Constant1/1 -> Create diagonal 3x3 matrix/1(Vector)
  Create diagonal 3x3 matrix/1(Matrix) -> Product1/2
  Product/1 -> Out1/1

== system Sim_Multi/State Estimation, Sensors, Noise/State estimation/Normalize/norm/dot_product ==
  u : Inport
  v : Inport  Port=2
  Product : Product  Multiplication=Matrix(*)  RndMeth=Zero
  Reshape : Reshape  OutputDimensionality=Column vector (2-D)
  Reshape1 : Reshape  OutputDimensionality=Column vector (2-D)
  transpose : Math  Operator=transpose  SignedPower=on
  u.v : Outport
  wires:
  v/1 -> Reshape1/1
  u/1 -> Reshape/1
  Reshape/1 -> transpose/1
  transpose/1 -> Product/1
  Reshape1/1 -> Product/2
  Product/1 -> u.v/1

== system Sim_Multi/multirotor/6DOF model/Calculate omega_dot/Cross Product omega x (J * omega)/Subsystem ==
  u : Inport
  v : Inport  Port=2
  Demux : Demux  Outputs=3
  Demux1 : Demux  Outputs=3
  Mux : Mux  Inputs=3
  Product : Product
  Product1 : Product
  Product2 : Product
  Positive elements : Outport
  wires:
  Mux/1 -> Positive elements/1
  v/1 -> Demux1/1
  u/1 -> Demux/1
  Demux/2 -> Product/1
  Demux1/3 -> Product/2
  Demux/3 -> Product1/1
  Demux1/1 -> Product1/2
  Demux/1 -> Product2/1
  Demux1/2 -> Product2/2
  Product/1 -> Mux/1  "u2*v3"
  Product1/1 -> Mux/2  "u3*v1"
  Product2/1 -> Mux/3  "u1*v2"

== system Sim_Multi/multirotor/6DOF model/Calculate omega_dot/Cross Product omega x (J * omega)/Subsystem1 ==
  u : Inport
  v : Inport  Port=2
  Demux : Demux  Outputs=3
  Demux1 : Demux  Outputs=3
  Mux : Mux  Inputs=3
  Product : Product
  Product1 : Product
  Product2 : Product
  Negative elements : Outport
  wires:
  Mux/1 -> Negative elements/1
  v/1 -> Demux1/1
  u/1 -> Demux/1
  Product/1 -> Mux/1  "u3*v2"
  Product1/1 -> Mux/2  "u1*v3"
  Product2/1 -> Mux/3  "u2*v1"
  Demux/3 -> Product/1
  Demux1/2 -> Product/2
  Demux/1 -> Product1/1
  Demux1/3 -> Product1/2
  Demux/2 -> Product2/1
  Demux1/1 -> Product2/2

== system Sim_Multi/multirotor/6DOF model/Quat Strapdown Eq./Cross Product/Subsystem ==
  u : Inport
  v : Inport  Port=2
  Demux : Demux  Outputs=3
  Demux1 : Demux  Outputs=3
  Mux : Mux  Inputs=3
  Product : Product
  Product1 : Product
  Product2 : Product
  Positive elements : Outport
  wires:
  Mux/1 -> Positive elements/1
  v/1 -> Demux1/1
  u/1 -> Demux/1
  Demux/2 -> Product/1
  Demux1/3 -> Product/2
  Demux/3 -> Product1/1
  Demux1/1 -> Product1/2
  Demux/1 -> Product2/1
  Demux1/2 -> Product2/2
  Product/1 -> Mux/1  "u2*v3"
  Product1/1 -> Mux/2  "u3*v1"
  Product2/1 -> Mux/3  "u1*v2"

== system Sim_Multi/multirotor/6DOF model/Quat Strapdown Eq./Cross Product/Subsystem1 ==
  u : Inport
  v : Inport  Port=2
  Demux : Demux  Outputs=3
  Demux1 : Demux  Outputs=3
  Mux : Mux  Inputs=3
  Product : Product
  Product1 : Product
  Product2 : Product
  Negative elements : Outport
  wires:
  Mux/1 -> Negative elements/1
  v/1 -> Demux1/1
  u/1 -> Demux/1
  Product/1 -> Mux/1  "u3*v2"
  Product1/1 -> Mux/2  "u1*v3"
  Product2/1 -> Mux/3  "u2*v1"
  Demux/3 -> Product/1
  Demux1/2 -> Product/2
  Demux/1 -> Product1/1
  Demux1/3 -> Product1/2
  Demux/2 -> Product2/1
  Demux1/1 -> Product2/2

== system Sim_Multi/multirotor/6DOF model/Quat Strapdown Eq./Normalize/norm ==
  u : Inport
  Complex to Real-Imag : ComplexToRealImag  Output=Real
  Sqrt : Sqrt
  dot_product : Subsystem
  ||u|| : Outport
  wires:
  u/1 -> dot_product/1(u), dot_product/2(v)
  dot_product/1(u.v) -> Sqrt/1
  Sqrt/1 -> Complex to Real-Imag/1
  Complex to Real-Imag/1 -> ||u||/1

== system Sim_Multi/multirotor/Force//Moment computation/Compute aerodynamic drag of the airframe in Body axes/Aerodynamic drag force/Nonzero airspeed ==
  Airspeed (Body) : Inport
  Surface_params : Inport  Port=2
  Action Port : ActionPort  ActionPortLabel=else
  Abs : Abs  SaturateOnIntegerOverflow=off
  Constant : Constant  Value=1/2
  Constant1 : Constant  Value=rho
  Constant2 : Constant  Value=C_D
  Drag force opposes direction of airspeed : Gain  Gain=-1
  Normalize : Subsystem
  Product : Product  Inputs=5
  Product1 : Product
  Surface area computation : Subsystem
  u^2 : Subsystem
  Drag force : Outport
  wires:
  Airspeed (Body)/1 -> Surface area computation/1(Airspeed (Body)), Normalize/1(Input), u^2/1(u)
  Surface_params/1 -> Surface area computation/2(Surface_params)
  Constant/1 -> Product/1
  Constant1/1 -> Product/2
  u^2/1(u^2) -> Product/3
  Constant2/1 -> Product/4
  Surface area computation/1(Area) -> Product/5
  Normalize/1(Output) -> Product1/1  "Normalized airspeed vector (Body axes)"
  Product1/1 -> Drag force opposes direction of airspeed/1
  Drag force opposes direction of airspeed/1 -> Drag force/1
  Product/1 -> Abs/1
  Abs/1 -> Product1/2  "Magnitude of drag force"

== system Sim_Multi/multirotor/Force//Moment computation/Compute aerodynamic drag of the airframe in Body axes/Aerodynamic drag force/Zero airspeed ==
  Airspeed : Inport
  Surface_params : Inport  Port=2
  Action Port : ActionPort  ActionPortLabel=if(u1 == 0)
  Constant : Constant  Value=[0;0;0]
  Terminator : Terminator
  Terminator1 : Terminator
  Drag force : Outport  InitialOutput=[0;0;-1]
  wires:
  Airspeed/1 -> Terminator/1  "Airspeed components in (unbent) rotor plane"
  Constant/1 -> Drag force/1
  Surface_params/1 -> Terminator1/1

== system Sim_Multi/multirotor/Force//Moment computation/Compute aerodynamic drag of the airframe in Body axes/Aerodynamic drag force/norm ==
  u : Inport
  Complex to Real-Imag : ComplexToRealImag  Output=Real
  Sqrt : Sqrt
  dot_product : Subsystem
  ||u|| : Outport
  wires:
  u/1 -> dot_product/1(u), dot_product/2(v)
  dot_product/1(u.v) -> Sqrt/1
  Sqrt/1 -> Complex to Real-Imag/1
  Complex to Real-Imag/1 -> ||u||/1

== system Sim_Multi/multirotor/Force//Moment computation/Compute aerodynamic drag of the airframe in Body axes/Total airspeed (Body axes)/Inertial to Body ==
  DCM_ib : Inport
  Wind_i : Inport  Port=2
  Product : Product  Multiplication=Matrix(*)
  Reshape : Reshape  OutputDimensionality=Column vector (2-D)
  Reshape1 : Reshape  OutputDimensionality=Column vector (2-D)
  Wind_b : Outport
  wires:
  Reshape/1 -> Product/2
  Product/1 -> Reshape1/1
  Reshape1/1 -> Wind_b/1
  Wind_i/1 -> Reshape/1
  DCM_ib/1 -> Product/1  "DCM_ib"

== system Sim_Multi/multirotor/Force//Moment computation/Forces and moments generated by spinning propellers/For Each Subsystem/Actuator dynamics ==
  note: This block diagram expresses the actuator dynamics of a specific motor/propeller combination
      | as a first order transfer function. The time constant and gain of this first order transfer function
      | for each motor is listed in the motor matrix.
      | In addition, upper and lower limits of the motor RPM can be set so that the motor output
      | never exceeds those values.
  MotorMatrix_real : Inport
  RPM_command : Inport  Port=2
  Continuous Integrator with dynamic upper/lower limits : Subsystem
  Continuous Integrator with dynamic upper/lower limits1 : Subsystem
  Divide : Product  Inputs=*/
  Product : Product  RndMeth=Zero  SampleTime=t_sim
  Selector : Selector  InputPortWidth=17  IndexOptions=Index vector (dialog)  Indices=[5]  OutputSizes=1
  Selector1 : Selector  InputPortWidth=17  IndexOptions=Index vector (dialog)  Indices=[6]  OutputSizes=1
  Selector2 : Selector  InputPortWidth=17  IndexOptions=Index vector (dialog)  Indices=[11]  OutputSizes=1
  Selector3 : Selector  InputPortWidth=17  IndexOptions=Index vector (dialog)  Indices=[12]  OutputSizes=1
  Sum1 : Sum  Inputs=-+|
  RPM_motor : Outport
  wires:
  Sum1/1 -> Divide/1
  Selector1/1 -> Divide/2  "TF time constant"
  Product/1 -> Sum1/2
  Selector/1 -> Product/2  "TF gain"
  RPM_command/1 -> Product/1
  MotorMatrix_real/1 -> Selector3/1, Selector2/1, Selector1/1, Selector/1
  Divide/1 -> Continuous Integrator with dynamic upper/lower limits/1(Integrator input)
  Continuous Integrator with dynamic upper/lower limits/1(Output) -> RPM_motor/1, Sum1/1
  Selector2/1 -> Continuous Integrator with dynamic upper/lower limits/2(Lower limit)  "RPM min value"
  Selector3/1 -> Continuous Integrator with dynamic upper/lower limits/3(Upper limit)  "RPM max value"

== system Sim_Multi/multirotor/Force//Moment computation/Forces and moments generated by spinning propellers/For Each Subsystem/Cross Product ==
  r : Inport
  omega : Inport  Port=2
  Reshape : Reshape  OutputDimensionality=Column vector (2-D)
  Subsystem : Subsystem
  Subsystem1 : Subsystem
  Sum : Sum  Inputs=+|-
  omega x r : Outport
  wires:
  Sum/1 -> Reshape/1
  omega/1 -> Subsystem1/1(omega), Subsystem/1(omega)
  r/1 -> Subsystem1/2(r), Subsystem/2(r)
  Subsystem/1(Positive elements) -> Sum/1
  Subsystem1/1(Negative elements) -> Sum/2
  Reshape/1 -> omega x r/1
